simulink model "MPPT_eolo"  (R2021a)
settings: Solver=VariableStepAuto  StartTime=0.0  StopTime=5.5  RelTol=1e-3
model workspace (MAT data in the model file):
  x = 50
libraries: spsDiodeLib x7, spsSeriesRLCBranchLib x4, spsCurrentMeasurementLib x2, spsVoltageMeasurementLib x2, spsPWMGeneratorDCDCLib x1, spsGroundLib x1, spsMosfetLib x1, spsPermanentMagnetSynchronousMachineLib x1, spspowerguiLib x1
settings Model: Creator=root  LastModifiedBy=Victor
settings SolverCC: AlgebraicLoopSolver=TrustRegion
settings DebuggingCC: SFMachineParentedDataDiag=warning

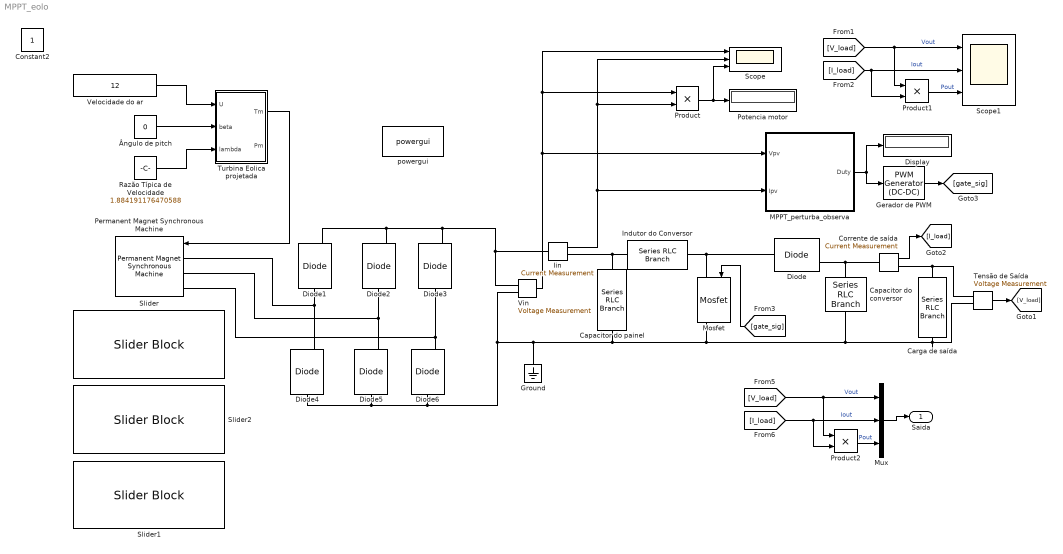
== system MPPT_eolo ==
  Capacitor do conversor : spsSeriesRLCBranchLib/Series RLC Branch  LConnTagsString=__new0  RConnTagsString=__new0  BranchType=C  Resistance=1e-4  Inductance=1e-3  SetiL0=off  InitialCurrent=0  Capacitance=2200e-6  Setx0=off  InitialVoltage=0  Measurements=None
  Capacitor do painel : spsSeriesRLCBranchLib/Series RLC Branch  LConnTagsString=__new0  RConnTagsString=__new0  BranchType=C  Resistance=1e-4  Inductance=1e-3  SetiL0=off  InitialCurrent=0  Capacitance=4700e-6  Setx0=off  InitialVoltage=0  Measurements=None
  "Carga de saída " : spsSeriesRLCBranchLib/Series RLC Branch  LConnTagsString=__new0  RConnTagsString=__new0  BranchType=R  Resistance=10  Inductance=1e-3  SetiL0=off  InitialCurrent=0  Capacitance=20e-6  Setx0=off  InitialVoltage=0  Measurements=None
  Corrente de saída : spsCurrentMeasurementLib/Current Measurement  PhasorSimulation=off  OutputType=Complex  PSBequivalent=0
  Diode{,1..6} (7 alike) : spsDiodeLib/Diode  Ron=0.001  Lon=0  Vf=0.8  IC=0  UseSnubber=0  Rs=500  Cs=250e-9  Measurements=on
  Display : Display
  Gerador de PWM : spsPWMGeneratorDCDCLib/PWM Generator (DC-DC)  Fsw=5e3  Ts=0
  Ground : spsGroundLib/Ground  LConnTagsString=a
  Iin : spsCurrentMeasurementLib/Current Measurement  PhasorSimulation=off  OutputType=Complex  PSBequivalent=0
  Indutor do Conversor : spsSeriesRLCBranchLib/Series RLC Branch  LConnTagsString=__new0  RConnTagsString=__new0  BranchType=L  Resistance=1e-4  Inductance=3400e-6  SetiL0=off  InitialCurrent=0  Capacitance=100e-6  Setx0=off  InitialVoltage=0  Measurements=None
  MPPT_perturba_observa : MATLAB Function  TreatAsAtomicUnit=on
  Mosfet : spsMosfetLib/Mosfet  Ron=0.1  Lon=0  Rd=0.01  Vfd=0  IC=0  Rs=1e5  Cs=inf  Measurements=on
  Mux : Mux  Inputs=3
  Permanent Magnet Synchronous Machine : spsPermanentMagnetSynchronousMachineLib/Permanent Magnet Synchronous Machine  NbPhases=3  FluxDistribution=Sinusoidal  RotorType=Round  MechanicalLoad=Torque Tm  PresetModel=No  ShowDetailedParameters=on  MeasurementBus=off  Resistance=0.001  Inductance=8.5e-3  dqInductances=[8.5e-3,8.5e-3]  La=0.00001365  MachineConstant=Voltage Constant (V_peak L-L / krpm)  Flux=0.088213  VoltageCst=96  TorqueCst=0.79391  Flat=120  Mechanical=[0.0001 0.01 6 10]  PolePairs=4  InitialConditions=[0,0, 0,0]  InitialConditions5ph=[0 0 0 0 0 0]  RefAngle=Aligned with phase A axis (original Park)  IterativeDiscreteModel=Trapezoidal non iterative  TsBlock=-1  TsPowergui=0
  Potencia motor : Display
  Product : Product
  Product1 : Product
  Product2 : Product
  Razão Típica de Velocidade : Constant  Value=1.884191176470588
  Scope : Scope  NumInputPorts=3
  Scope1 : Scope  NumInputPorts=3
  Slider : SliderBlock  ScaleMax=12
  Slider1 : SliderBlock  ScaleMax=10
  Slider2 : SliderBlock  ScaleMax=5
  Tensão de Saída : spsVoltageMeasurementLib/Voltage Measurement  PhasorSimulation=off  OutputType=Complex  PSBequivalent=0
  Turbina Eolica projetada : Subsystem
  Velocidade do ar : Constant  Value=12
  Vin : spsVoltageMeasurementLib/Voltage Measurement  PhasorSimulation=off  OutputType=Complex  PSBequivalent=0
  powergui : spspowerguiLib/powergui  Priority=1  SimulationMode=Discrete  SampleTime=1e-6  frequency=60  Iterations=50  frequencyindice=0  Pbase=100e6  ErrMax=1e-4  UnitsV=kV  UnitsW=MW  buscounter=0  FunctionMessages=off  echomessages=off  EnableUseOfTLC=off  CurrentSourceSwitches=off  DisableSnubberDevices=off  DisableRonSwitches=off  DisableVfSwitches=off  DisplayEquations=off  AutomaticDiscreteSolvers=off  SolverType=Tustin/Backward Euler (TBE)  Interpol=off  ExternalGateDelay=off  methode=off  Ts=100  x0status=blocks  SPID=on  SwTol=0  HookPort=off  NonlinearTolerance=1e-4  nMaxIteration=100  ContinueOnMaxIteration=off  RestoreLinks=warning  ResistiveCurrentMeasurement=off  Frange=[0:2:500]  Ylog=off  Xlog=on  ShowGrid=off  save=off  variable=ZData  structure=0  ZoomFFT=off  StartTime=0.0  cycles=1  DisplayStyle=1  fundamental=60  FreqAxis=off  MaxFrequency=1000  frequencyindicesteady=1  RmsSteady=1  display=off
  Ângulo de pitch : Constant  Value=0
  Saida : Outport
  Constant2 : Constant  IOType=siggen
  wires:
  Vin/1 -> Product/1, Scope/1, MPPT_perturba_observa/1(Vpv)
  Iin/1 -> Scope/2, Product/2, MPPT_perturba_observa/2(Ipv)
  Tensão de Saída/1 -> [V_load]
  Corrente de saída/1 -> [I_load]
  [V_load] -> Product1/1, Scope1/1  "Vout"
  [I_load] -> Scope1/2, Product1/2  "Iout"
  Gerador de PWM/1 -> [gate_sig]
  Product/1 -> Scope/3, Potencia motor/1
  MPPT_perturba_observa/1(Duty) -> Gerador de PWM/1, Display/1
  Product1/1 -> Scope1/3  "Pout"
  [gate_sig] -> Mosfet/1
  Mux/1 -> Saida/1
  [V_load] -> Product2/1, Mux/1  "Vout"
  [I_load] -> Mux/2, Product2/2  "Iout"
  Product2/1 -> Mux/3  "Pout"
  Velocidade do ar/1 -> Turbina Eolica projetada/1(U)
  Ângulo de pitch/1 -> Turbina Eolica projetada/2(beta)
  Razão Típica de Velocidade/1 -> Turbina Eolica projetada/3(lambda)
  Turbina Eolica projetada/1(Tm) -> Permanent Magnet Synchronous Machine/1
  connections:
  "Carga de saída "/LConn1 -- Corrente de saída/RConn1 -- Tensão de Saída/LConn1
  Corrente de saída/LConn1 -- Diode/RConn1 -- Capacitor do conversor/LConn1
  Mosfet/LConn1 -- Diode/LConn1 -- Indutor do Conversor/LConn1
  Diode4/RConn1 -- Permanent Magnet Synchronous Machine/LConn1 -- Diode1/LConn1
  Diode5/RConn1 -- Permanent Magnet Synchronous Machine/LConn2 -- Diode2/LConn1
  Diode6/RConn1 -- Permanent Magnet Synchronous Machine/LConn3 -- Diode3/LConn1
  Diode1/RConn1 -- Diode2/RConn1 -- Vin/LConn1 -- Iin/LConn1 -- Diode3/RConn1
  "Carga de saída "/RConn1 -- Tensão de Saída/LConn2 -- Capacitor do conversor/RConn1 -- Mosfet/RConn1 -- Capacitor do painel/RConn1 -- Ground/LConn1 -- Vin/LConn2 -- Diode4/LConn1 -- Diode5/LConn1 -- Diode6/LConn1
  Indutor do Conversor/RConn1 -- Iin/RConn1 -- Capacitor do painel/LConn1

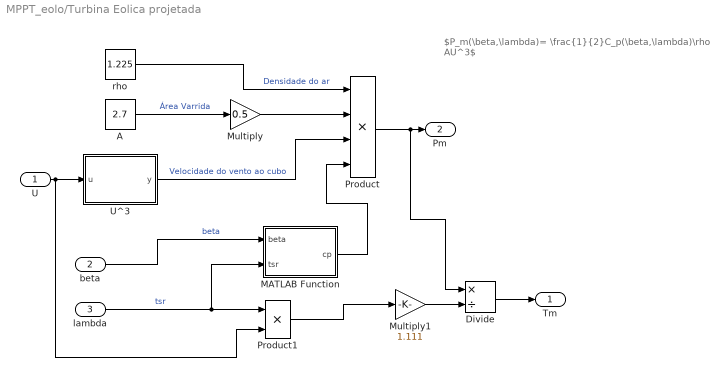
== system MPPT_eolo/Turbina Eolica projetada ==
  note: $P_m(\beta,\lambda)= \frac{1}{2}C_p(\beta,\lambda)\rho AU^3$
  U : Inport
  beta : Inport  Port=2
  lambda : Inport  Port=3
  A : Constant  Value=2.7
  Divide : Product  Inputs=*/
  MATLAB Function : MATLAB Function  TreatAsAtomicUnit=on
  Multiply : Gain  Gain=0.5
  Multiply1 : Gain  Gain=1.111
  Product : Product  Inputs=4
  Product1 : Product
  U^3 : MATLAB Function  TreatAsAtomicUnit=on
  rho : Constant  Value=1.225
  Tm : Outport
  Pm : Outport  Port=2
  wires:
  Product/1 -> Divide/1, Pm/1
  A/1 -> Multiply/1  "Área Varrida"
  Multiply/1 -> Product/2
  rho/1 -> Product/1  "Densidade do ar"
  U/1 -> Product1/2, U^3/1(u)
  U^3/1(y) -> Product/3  "Velocidade do vento ao cubo"
  beta/1 -> MATLAB Function/1(beta)  "beta"
  MATLAB Function/1(cp) -> Product/4
  lambda/1 -> Product1/1, MATLAB Function/2(tsr)  "tsr"
  Product1/1 -> Multiply1/1
  Multiply1/1 -> Divide/2
  Divide/1 -> Tm/1

== matlab function MPPT_eolo/Turbina Eolica projetada/U^3 ==
  data: u input; y output
function y = fcn(u)
y = u^3;

== matlab function MPPT_eolo/Turbina Eolica projetada/MATLAB Function ==
  data: beta input; cp output; tsr input
function cp = fcn(beta, tsr)
c1 = 0.387;
c2 = 116;
c3 = 0.4;
c4 = 5;
c5 = 21;
c6 = 0.08;
c7 = 0.035;
c8 = 0.00413;
c9 = 3.7;
cp = c1*((-c4-c3*(2.5+beta)+c2/(c9*tsr+c6*(2.5+beta)) -c2*c7/(c9*tsr+(2.5+beta)^3))/exp(c5*(1/(c9*tsr+c6*(2.5+beta))-c7/(c9*tsr+(2.5+beta)^3)))) + c8*c9*tsr;

== matlab function MPPT_eolo/MPPT_perturba_observa ==
  data: Vpv input; Duty output; Ipv input
function Duty = MPPT_perturba_observa(Vpv, Ipv)


    %% Declaração das variaveis como persistent de forma que os valores 
    %  fiquem armazenados mesmo com o término da função
    
    persistent Vpv_old Ppv_old Duty_old
    
    % Inicializacao das variaveis
    if isempty(Duty_old)
       Duty_old = 0.5;
       Ppv_old = 0;
       Vpv_old = 0;
    end
    
    Duty_var = 100e-6;           % Delta de variacao a cada iteracao
    
    
    % Calculo do valor de potencia
    
    Ppv = Vpv * Ipv;
    
    %% Inicializacao da comparacao
    
    if ((Ppv - Ppv_old) ~= 0)
       if ((Ppv - Ppv_old) < 0) 
            if ((Vpv - Vpv_old) < 0)
                Duty = Duty_old - Duty_var;
            else 
                Duty = Duty_old + Duty_var;
            end
       else 
           if ((Vpv - Vpv_old) < 0)
                Duty = Duty_old + Duty_var;
           else 
               Duty = Duty_old - Duty_var;
           end
       end
    else 
        
        Duty = Duty_old;
        
    end
    
    if (Duty > 1)
        Duty = 1.0;
    elseif Duty < 0
        Duty = 0.0;
    end 
    
    Ppv_old = Ppv;
    Vpv_old = Vpv;
    Duty_old = Duty;    
end
